simulink model "AxialPump_23a"  (R2023a)
settings: Solver=FixedStepAuto  StartTime=0.0  StopTime=t_cycle  FixedStep=1e-8  RelTol=1e-3  EnableMultiTasking=on
InitFcn:
  | %% Outlet
  | % Parameters
  | d_cyl = 8e-3;                                   % Diameter of each piston
  | r_p = 20e-3;                                    % Piston pitch radius
  | A_cyl = 0.25 * pi * d_cyl^2;                    % Area of each piston
  | omega_rpm = 3600;                               % Rotational speed of pump
  | omega = (2*pi/60) * omega_rpm;                  % Angular speed of pump
  | beta = 1.6e9;                                   % Bulk Modulus
  | P1 = 21e6;                                      % Outlet pressure
  | S = 15e-3;                                      % Stroke length
  | Cd = 0.6;                                       % Coefficient of discharge
  | rho = 870;                                      % Density
  | P_T = 101325;                                   % Tank pressure
  | P_P = 21e6;                                     % System pressure
  | c = 80e-6;                                      % Piston-barrel clearance
  | meu = 0.1;                                      % Steel-steel (lubricated) coefficient of friction
  | r2_r1 = 1.6;                                    % Slipper radii ratio
  | r1 = d_cyl/2;
  | do = 0.1e-3;                                    % Slipper orifice opening
  | 
  | % Time parameters
  | theta_cycle = 2 * pi;
  | t_cycle = theta_cycle / omega;
  | theta_t = 2 * asin(d_cyl/(4*r_p));
  | t_t = theta_t/omega;
  | theta_d = theta_cycle/2 - 2 * theta_t;
  | t_d = theta_d/omega;
  | 
  | t_A_p = [0, 0.5*t_t, t_t, t_t+t_d, 1.5*t_t+t_d, t_cycle];
  | A_p = [0, 0, A_cyl, A_cyl, 0, 0];
  | 
  | t_A_t = [0, 2.5*t_t+t_d, 3*t_t+t_d, 3*t_t+2*t_d, 3.5*t_t+2*t_d, t_cycle];
  | A_t = [0, 0, A_cyl, A_cyl, 0, 0];
  | 
  | % Calculated parameters
  | Vdisp = 0.25 * pi * d_cyl^2 * S;
  | Vo = Vdisp;
libraries: SignalEditorBlockLib x18
(part 1 of 2)
settings Model: Creator=user  LastModifiedBy=ibrah408
settings SolverCC: AutoInsertRateTranBlk=on
settings DataIOCC: SaveOutput=off  SaveTime=off
settings OptimizationCC: DefaultParameterBehavior=Inlined  InlineInvariantSignals=on  EnhancedBackFolding=on  PassReuseOutputArgsAs=Individual arguments  StateBitsets=on  DataBitsets=on  ZeroExternalMemoryAtStartup=off  ZeroInternalMemoryAtStartup=off  NoFixptDivByZeroProtection=on  LifeSpan=1  OptimizeBlockOrder=speed  DifferentSizesBufferReuse=on  EfficientTunableParamExpr=on
settings DebuggingCC: ParameterTunabilityLossMsg=error
settings HardwareCC: ProdBitPerPointer=32  ProdBitPerSizeT=32  ProdBitPerPtrDiffT=32  ProdLargestAtomicFloat=None  ProdIntDivRoundTo=Floor  ProdWordSize=32  ProdHWDeviceType=Generic->Custom
settings SFSimCC: MATLABDynamicMemAlloc=off
settings RTWCC: Description=Embedded Coder  SystemTargetFile=ert.tlc  TLCOptions=-p0  GenCodeOnly=on  TemplateMakefile=ert_default_tmf  GenerateReport=on  RTWVerbose=off  IncludeHyperlinkInReport=on  LaunchReport=on
settings CodeAppCC: ForceParamTrailComments=on  IgnoreCustomStorageClasses=off  OperatorAnnotations=on  SimulinkDataObjDesc=on  SFDataObjDesc=on  CustomSymbolStrGlobalVar=rt$N$M  CustomSymbolStrType=$N$M  CustomSymbolStrFcn=$N$M$F  CustomSymbolStrMacro=$N$M  InsertBlockDesc=on
settings ERTTargetCC: TargetLangStandard=C99 (ISO)  CodeReplacementLibrary=ISO_C  GenerateSampleERTMain=on  IncludeMdlTerminateFcn=off  SuppressErrorStatus=on  SupportAbsoluteTime=off  PurelyIntegerCode=on  SupportNonFinite=off  SupportComplex=off  InlinedParameterPlacement=NonHierarchical  RootIOFormat=Structure reference  ERTCustomFileTemplate=example_file_process.tlc

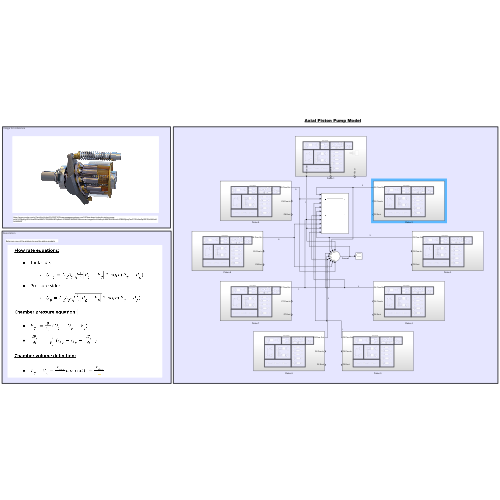
[thumbnail: Simulink's stored preview of the top-level diagram]
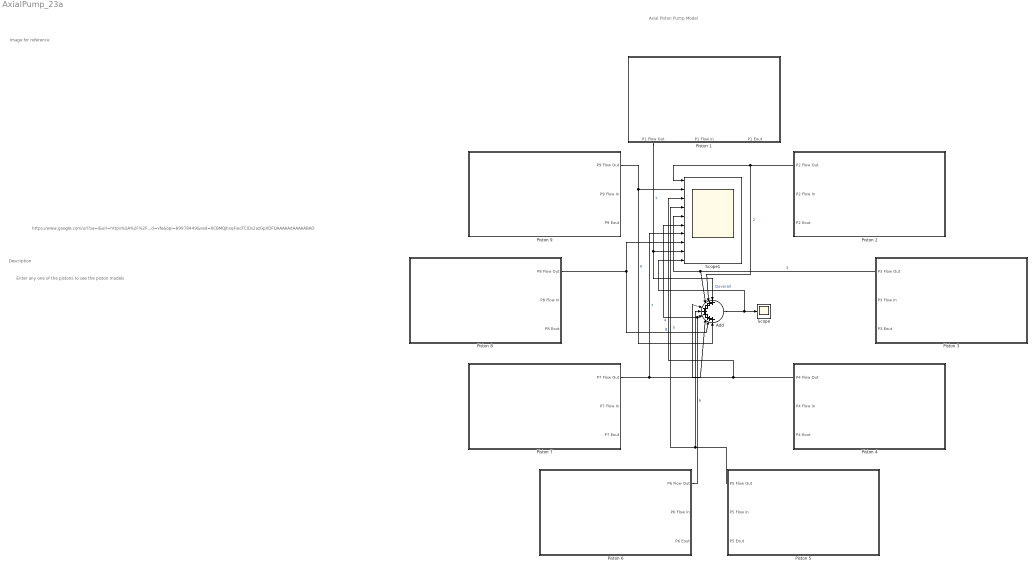
== system AxialPump_23a ==
  note: https://www.google.com/url?sa=i&url=https%3A%2F%2Fwww.panagonsystems.com%2Fhow-does-hydraulic-piston-pump-work%2F&psig=AOvVaw3SHzdt8MCUTcQAiBkLNfYq&ust=1698988184504000&source=images&cd=vfe&opi=89978449&ved=0CBMQjhxqFwoTCIDs2azGpIIDFQAAAAAdAAAAABAD
  note: Enter any one of the pistons to see the piston models
  note: Description
  note: Image for reference
  note: Axial Piston Pump Model
  Add : Sum  Inputs=+++++++++
  Piston 1 : Subsystem
      settings: PortSchema="{\"entries\":[{\"content\":{\"sides\":[{\"content\":{},\"type\":\"ConnectorPlacement.EquallySpacedRectSide\",\"uuid\":\"63442bf7-0830-4237-9a0b-f9adcef68f77\"},{\"content\":{\"side\":\"RIGHT\"},\"type\":\"ConnectorPlacement.EquallySpacedRectSide\",\"uuid\":\"c78b6823-6588-400d-8e0d-405a7015a902\"},{\"content\":{\"side\":\"TOP\"},\"type\":\"ConnectorPlacement.EquallySpacedRectSide\",\"uuid\":\"cf447a47-df1d-44f3-9a90-4edf3edff747\"},{\"content\":{\"connectorIds\":[\"Out1\",\"Out2\",\"Out3\"],\"side\":\"BOTTOM\"},\"type\":\"ConnectorPlacement.EquallySpacedRectSide\",\"uuid\":\"be505e56-dc88-4cf5-89cd-0d030a778f3c\"}]},\"type\":\"ConnectorPlacement.EquallySpacedConnector\",\"uuid\":\"51a26e02-629a-4264-944b-dee0710ca6c7\"}],\"packageUris\":[\"http://schema.mathworks.com/mf0/Connector/R2020b\"],\"version\":\"1.0\"}"
  Piston 2 : Subsystem
  Piston 3 : Subsystem
  Piston 4 : Subsystem
  Piston 5 : Subsystem
  Piston 6 : Subsystem
  Piston 7 : Subsystem
  Piston 8 : Subsystem
  Piston 9 : Subsystem
  Scope : Scope
  Scope1 : Scope  NumInputPorts=10
  wires:
  Add/1 -> Scope1/10, Scope/1  "Qoverall"
  Piston 2/1(P2 Flow Out) -> Scope1/1, Add/2  "2"
  Piston 3/1(P3 Flow Out) -> Scope1/5, Add/3  "3"
  Piston 4/1(P4 Flow Out) -> Scope1/3, Add/4  "4"
  Piston 5/1(P5 Flow Out) -> Add/5, Scope1/4  "5"
  Piston 6/1(P6 Flow Out) -> Scope1/6, Add/6  "6"
  Piston 7/1(P7 Flow Out) -> Scope1/7, Add/7  "7"
  Piston 8/1(P8 Flow Out) -> Add/8, Scope1/8  "8"
  Piston 9/1(P9 Flow Out) -> Add/9, Scope1/2  "9"
  Piston 1/1(P1 Flow Out) -> Add/1, Scope1/9  "1"

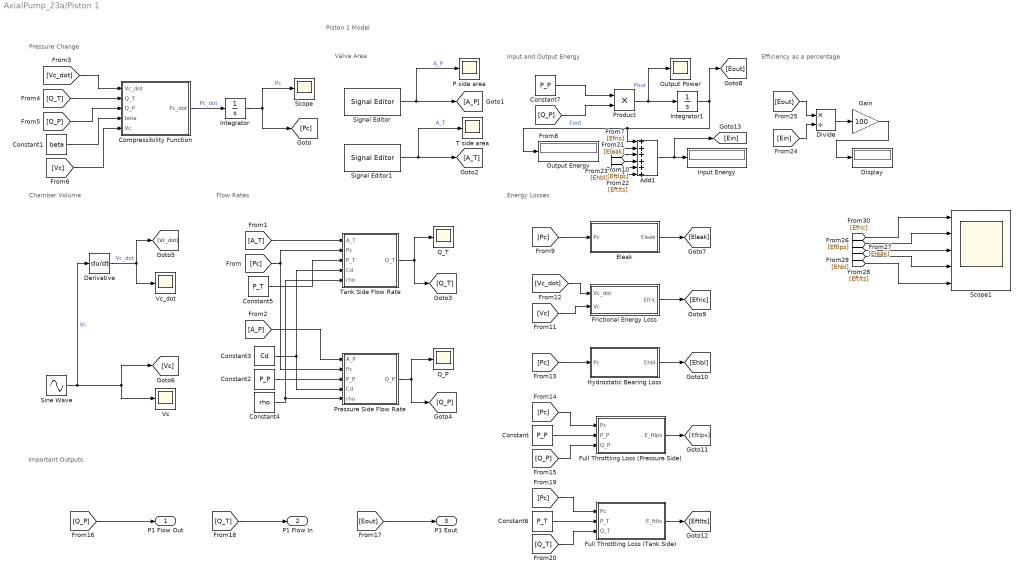
== system AxialPump_23a/Piston 1 ==
  note: Efficiency as a percentage
  note: Important Outputs
  note: Energy Losses
  note: Input and Output Energy
  note: Pressure Change
  note: Chamber Volume
  note: Valve Area
  note: Flow Rates
  note: Piston 1 Model
      | ​
  Add1 : Sum  Inputs=++++++
  Compressibility Function : MATLAB Function  TreatAsAtomicUnit=on
  Constant : Constant  Value=P_P
  Constant1 : Constant  Value=beta
  Constant2 : Constant  Value=P_P
  Constant3 : Constant  Value=Cd
  Constant4 : Constant  Value=rho
  Constant5 : Constant  Value=P_T
  Constant6 : Constant  Value=P_T
  Constant7 : Constant  Value=P_P
  Derivative : Derivative
  Display : Display
  Divide : Product  Inputs=*/
  Eleak : Subsystem
  Frictional Energy Loss : Subsystem
  Full Throttling Loss (Pressure Side) : Subsystem
  Full Throttling Loss (Tank Side) : Subsystem
  Gain : Gain  Gain=100
  Hydrostatic Bearing Loss : Subsystem
  Input Energy : Display
  Integrator : Integrator  InitialCondition=-2.0291e6  LowerSaturationLimit=0
  Integrator1 : Integrator
  Output Energy : Display
  Output Power : Scope
  P side area : Scope
  Pressure Side Flow Rate : MATLAB Function  TreatAsAtomicUnit=on
  Product : Product
  Q_P : Scope
  Q_T : Scope
  Scope : Scope
  Scope1 : Scope  NumInputPorts=5
  Signal Editor : SignalEditorBlockLib/Signal Editor  FileName=A_P.mat  ActiveScenario=Scenario  ActiveSignal=A_P  IsBus=off  OutputBusObjectStr=Bus: BusObject  SampleTime=0  ZeroCross=off  OutputAfterFinalValue=Setting to zero  Unit=inherit  PreserveSignalName=on  ApplySigPropsToAllScenarios=on
  Signal Editor1 : SignalEditorBlockLib/Signal Editor  FileName=A_T.mat  ActiveScenario=Scenario  ActiveSignal=A_T  IsBus=off  OutputBusObjectStr=Bus: BusObject  SampleTime=0  ZeroCross=off  OutputAfterFinalValue=Setting to zero  Unit=inherit  PreserveSignalName=on  ApplySigPropsToAllScenarios=on
  Sine Wave : Sin  Amplitude=Vdisp/2  Bias=Vo + (Vdisp/2)  Frequency=omega  Phase=pi/2  SampleTime=0
  T side area : Scope
  Tank Side Flow Rate : MATLAB Function  TreatAsAtomicUnit=on
  Vc : Scope
  Vc_dot : Scope
  P1 Flow Out : Outport
  P1 Flow In : Outport  Port=2
  P1 Eout : Outport  Port=3
  wires:
  Signal Editor/1 -> P side area/1, [A_P]  "A_P"
  [Pc] -> Hydrostatic Bearing Loss/1(Pc)
  [A_P] -> Pressure Side Flow Rate/1(A_P)
  [Pc] -> Full Throttling Loss (Pressure Side)/1(Pc)
  [Q_P] -> Full Throttling Loss (Pressure Side)/3(Q_P)
  Constant/1 -> Full Throttling Loss (Pressure Side)/2(P_P)
  Pressure Side Flow Rate/1(Q_P) -> Q_P/1, [Q_P]
  Tank Side Flow Rate/1(Q_T) -> Q_T/1, [Q_T]
  Constant4/1 -> Tank Side Flow Rate/5(rho), Pressure Side Flow Rate/5(rho)
  Constant2/1 -> Pressure Side Flow Rate/3(P_P)
  [Q_P] -> Compressibility Function/3(Q_P)
  Signal Editor1/1 -> [A_T], T side area/1  "A_T"
  [A_T] -> Tank Side Flow Rate/1(A_T)
  Constant1/1 -> Compressibility Function/4(beta)
  [Pc] -> Pressure Side Flow Rate/2(Pc), Tank Side Flow Rate/2(Pc)
  [Vc_dot] -> Compressibility Function/1(Vc_dot)
  [Q_T] -> Compressibility Function/2(Q_T)
  Compressibility Function/1(Pc_dot) -> Integrator/1  "Pc_dot"
  [Vc] -> Compressibility Function/5(Vc)
  Sine Wave/1 -> [Vc], Vc/1, Derivative/1  "Vc"
  Integrator/1 -> [Pc], Scope/1  "Pc"
  Constant3/1 -> Tank Side Flow Rate/4(Cd), Pressure Side Flow Rate/4(Cd)
  Derivative/1 -> Vc_dot/1, [Vc_dot]  "Vc_dot"
  Constant5/1 -> Tank Side Flow Rate/3(P_T)
  [Vc_dot] -> Frictional Energy Loss/1(Vc_dot)
  [Vc] -> Frictional Energy Loss/2(Vc)
  [Q_P] -> P1 Flow Out/1
  [Eout] -> P1 Eout/1
  [Q_T] -> P1 Flow In/1
  [Pc] -> Full Throttling Loss (Tank Side)/1(Pc)
  Constant6/1 -> Full Throttling Loss (Tank Side)/2(P_T)
  [Q_T] -> Full Throttling Loss (Tank Side)/3(Q_T)
  Constant7/1 -> Product/1
  Product/1 -> Integrator1/1, Output Power/1  "Pout"
  Add1/1 -> [Ein], Input Energy/1
  Integrator1/1 -> Output Energy/1, Add1/1, [Eout]  "Eout"
  [Q_P] -> Product/2
  [Pc] -> Eleak/1(Pc)
  Eleak/1(Eleak) -> [Eleak]
  Frictional Energy Loss/1(Efric) -> [Efric]
  Hydrostatic Bearing Loss/1(Ehbl) -> [Ehbl]
  Full Throttling Loss (Tank Side)/1(" E_ftlts") -> [Eftlts]
  Full Throttling Loss (Pressure Side)/1(" E_ftlps") -> [Eftlps]
  [Efric] -> Add1/2
  [Eftlps] -> Add1/3
  [Eleak] -> Add1/4
  [Eftlts] -> Add1/5
  [Ehbl] -> Add1/6
  [Ein] -> Divide/2
  [Eout] -> Divide/1
  Divide/1 -> Gain/1
  Gain/1 -> Display/1
  [Efric] -> Scope1/1
  [Eftlps] -> Scope1/2
  [Eleak] -> Scope1/3
  [Eftlts] -> Scope1/4
  [Ehbl] -> Scope1/5

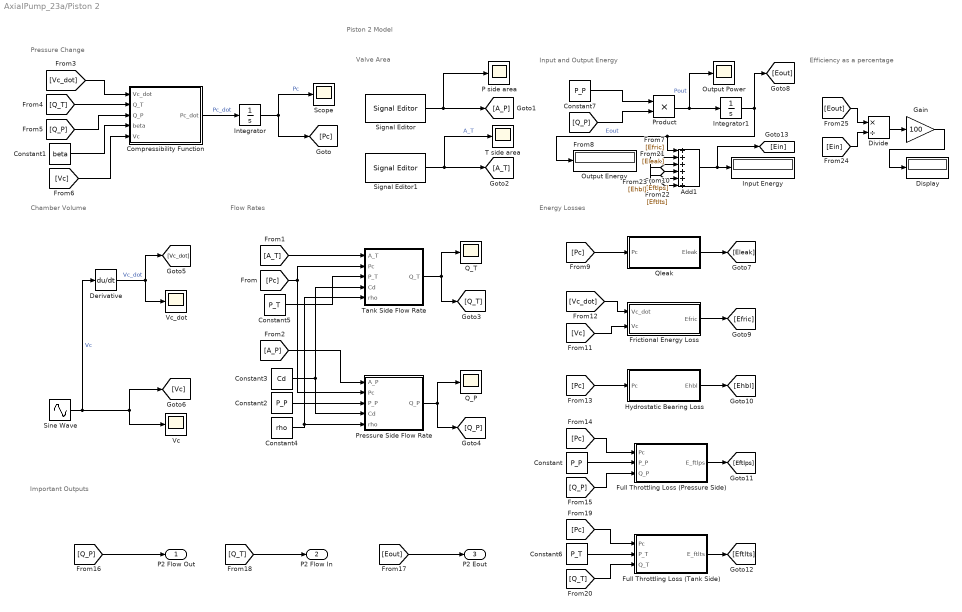
== system AxialPump_23a/Piston 2 ==
  note: Important Outputs
  note: Pressure Change
  note: Chamber Volume
  note: Valve Area
  note: Flow Rates
  note: Piston 2 Model
      | ​
  note: Energy Losses
  note: Efficiency as a percentage
  note: Input and Output Energy
  Add1 : Sum  Inputs=++++++
  Compressibility Function : MATLAB Function  TreatAsAtomicUnit=on
  Constant : Constant  Value=P_P
  Constant1 : Constant  Value=beta
  Constant2 : Constant  Value=P_P
  Constant3 : Constant  Value=Cd
  Constant4 : Constant  Value=rho
  Constant5 : Constant  Value=P_T
  Constant6 : Constant  Value=P_T
  Constant7 : Constant  Value=P_P
  Derivative : Derivative
  Display : Display
  Divide : Product  Inputs=*/
  Frictional Energy Loss : Subsystem
  Full Throttling Loss (Pressure Side) : Subsystem
  Full Throttling Loss (Tank Side) : Subsystem
  Gain : Gain  Gain=100
  Hydrostatic Bearing Loss : Subsystem
  Input Energy : Display
  Integrator : Integrator  InitialCondition=P_T
  Integrator1 : Integrator
  Output Energy : Display
  Output Power : Scope
  P side area : Scope
  Pressure Side Flow Rate : MATLAB Function  TreatAsAtomicUnit=on
  Product : Product
  Q_P : Scope
  Q_T : Scope
  Qleak : Subsystem
  Scope : Scope
  Signal Editor : SignalEditorBlockLib/Signal Editor  FileName=A_P_2.mat  ActiveScenario=Scenario  ActiveSignal=A_P_2  IsBus=off  OutputBusObjectStr=Bus: BusObject  SampleTime=0  ZeroCross=off  OutputAfterFinalValue=Setting to zero  Unit=inherit  PreserveSignalName=on  ApplySigPropsToAllScenarios=on
  Signal Editor1 : SignalEditorBlockLib/Signal Editor  FileName=A_T_2.mat  ActiveScenario=Scenario  ActiveSignal=A_T_2  IsBus=off  OutputBusObjectStr=Bus: BusObject  SampleTime=0  ZeroCross=off  OutputAfterFinalValue=Setting to zero  Unit=inherit  PreserveSignalName=on  ApplySigPropsToAllScenarios=on
  Sine Wave : Sin  Amplitude=Vdisp/2  Bias=Vo + (Vdisp/2)  Frequency=omega  Phase=pi/2-(2*pi/9)  SampleTime=0
  T side area : Scope
  Tank Side Flow Rate : MATLAB Function  TreatAsAtomicUnit=on
  Vc : Scope
  Vc_dot : Scope
  P2 Flow Out : Outport
  P2 Flow In : Outport  Port=2
  P2 Eout : Outport  Port=3
  wires:
  Signal Editor/1 -> P side area/1, [A_P]
  [A_P] -> Pressure Side Flow Rate/1(A_P)
  Pressure Side Flow Rate/1(Q_P) -> Q_P/1, [Q_P]
  Tank Side Flow Rate/1(Q_T) -> Q_T/1, [Q_T]
  Constant4/1 -> Tank Side Flow Rate/5(rho), Pressure Side Flow Rate/5(rho)
  Constant2/1 -> Pressure Side Flow Rate/3(P_P)
  [Q_P] -> Compressibility Function/3(Q_P)
  Signal Editor1/1 -> [A_T], T side area/1  "A_T"
  [A_T] -> Tank Side Flow Rate/1(A_T)
  Constant1/1 -> Compressibility Function/4(beta)
  [Pc] -> Pressure Side Flow Rate/2(Pc), Tank Side Flow Rate/2(Pc)
  [Vc_dot] -> Compressibility Function/1(Vc_dot)
  [Q_T] -> Compressibility Function/2(Q_T)
  Compressibility Function/1(Pc_dot) -> Integrator/1  "Pc_dot"
  [Vc] -> Compressibility Function/5(Vc)
  Sine Wave/1 -> [Vc], Vc/1, Derivative/1  "Vc"
  Integrator/1 -> [Pc], Scope/1  "Pc"
  Constant3/1 -> Tank Side Flow Rate/4(Cd), Pressure Side Flow Rate/4(Cd)
  Derivative/1 -> Vc_dot/1, [Vc_dot]  "Vc_dot"
  Constant5/1 -> Tank Side Flow Rate/3(P_T)
  [Q_P] -> P2 Flow Out/1
  [Eout] -> P2 Eout/1
  [Q_T] -> P2 Flow In/1
  [Pc] -> Qleak/1(Pc)
  [Eout] -> Divide/1
  Full Throttling Loss (Pressure Side)/1(" E_ftlps") -> [Eftlps]
  Full Throttling Loss (Tank Side)/1(" E_ftlts") -> [Eftlts]
  [Eftlts] -> Add1/5
  [Ehbl] -> Add1/6
  [Q_T] -> Full Throttling Loss (Tank Side)/3(Q_T)
  [Pc] -> Full Throttling Loss (Pressure Side)/1(Pc)
  [Pc] -> Full Throttling Loss (Tank Side)/1(Pc)
  [Vc] -> Frictional Energy Loss/2(Vc)
  [Vc_dot] -> Frictional Energy Loss/1(Vc_dot)
  [Pc] -> Hydrostatic Bearing Loss/1(Pc)
  Constant/1 -> Full Throttling Loss (Pressure Side)/2(P_P)
  [Q_P] -> Full Throttling Loss (Pressure Side)/3(Q_P)
  [Q_P] -> Product/2
  [Efric] -> Add1/2
  Constant6/1 -> Full Throttling Loss (Tank Side)/2(P_T)
  [Ein] -> Divide/2
  Divide/1 -> Gain/1
  Frictional Energy Loss/1(Efric) -> [Efric]
  Product/1 -> Integrator1/1, Output Power/1  "Pout"
  Constant7/1 -> Product/1
  Hydrostatic Bearing Loss/1(Ehbl) -> [Ehbl]
  Gain/1 -> Display/1
  Qleak/1(Eleak) -> [Eleak]
  Integrator1/1 -> Output Energy/1, Add1/1, [Eout]  "Eout"
  [Eftlps] -> Add1/3
  [Eleak] -> Add1/4
  Add1/1 -> [Ein], Input Energy/1

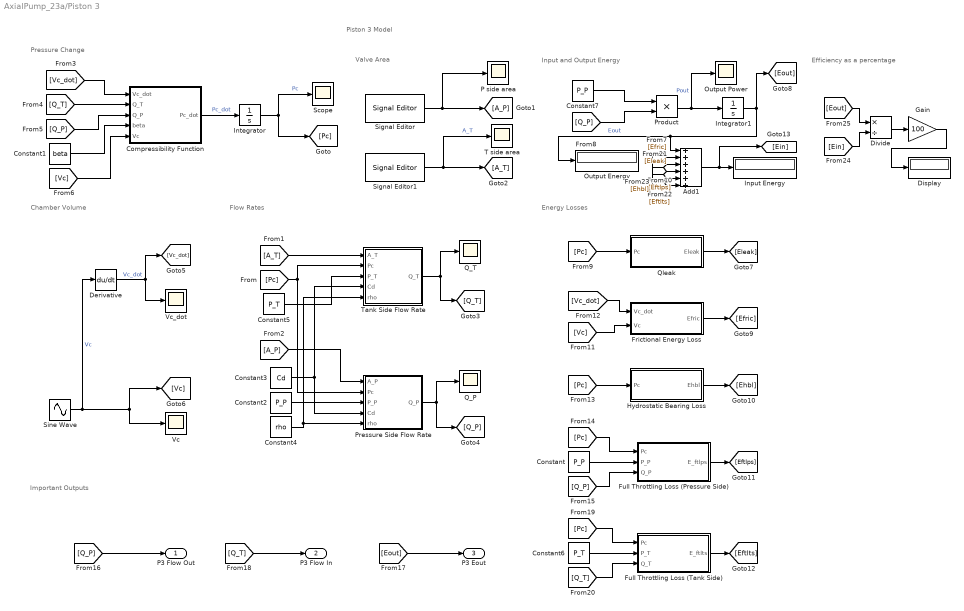
== system AxialPump_23a/Piston 3 ==
  note: Important Outputs
  note: Pressure Change
  note: Chamber Volume
  note: Valve Area
  note: Flow Rates
  note: Piston 3 Model
      | ​
  note: Energy Losses
  note: Efficiency as a percentage
  note: Input and Output Energy
  Add1 : Sum  Inputs=++++++
  Compressibility Function : MATLAB Function  TreatAsAtomicUnit=on
  Constant : Constant  Value=P_P
  Constant1 : Constant  Value=beta
  Constant2 : Constant  Value=P_P
  Constant3 : Constant  Value=Cd
  Constant4 : Constant  Value=rho
  Constant5 : Constant  Value=P_T
  Constant6 : Constant  Value=P_T
  Constant7 : Constant  Value=P_P
  Derivative : Derivative
  Display : Display
  Divide : Product  Inputs=*/
  Frictional Energy Loss : Subsystem
  Full Throttling Loss (Pressure Side) : Subsystem
  Full Throttling Loss (Tank Side) : Subsystem
  Gain : Gain  Gain=100
  Hydrostatic Bearing Loss : Subsystem
  Input Energy : Display
  Integrator : Integrator  InitialCondition=P_T
  Integrator1 : Integrator
  Output Energy : Display
  Output Power : Scope
  P side area : Scope
  Pressure Side Flow Rate : MATLAB Function  TreatAsAtomicUnit=on
  Product : Product
  Q_P : Scope
  Q_T : Scope
  Qleak : Subsystem
  Scope : Scope
  Signal Editor : SignalEditorBlockLib/Signal Editor  FileName=A_P_3.mat  ActiveScenario=Scenario  ActiveSignal=A_P_3  IsBus=off  OutputBusObjectStr=Bus: BusObject  SampleTime=0  ZeroCross=off  OutputAfterFinalValue=Setting to zero  Unit=inherit  PreserveSignalName=on  ApplySigPropsToAllScenarios=on
  Signal Editor1 : SignalEditorBlockLib/Signal Editor  FileName=A_T_3.mat  ActiveScenario=Scenario  ActiveSignal=A_T_3  IsBus=off  OutputBusObjectStr=Bus: BusObject  SampleTime=0  ZeroCross=off  OutputAfterFinalValue=Setting to zero  Unit=inherit  PreserveSignalName=on  ApplySigPropsToAllScenarios=on
  Sine Wave : Sin  Amplitude=Vdisp/2  Bias=Vo + (Vdisp/2)  Frequency=omega  Phase=pi/2-(4*pi/9)  SampleTime=0
  T side area : Scope
  Tank Side Flow Rate : MATLAB Function  TreatAsAtomicUnit=on
  Vc : Scope
  Vc_dot : Scope
  P3 Flow Out : Outport
  P3 Flow In : Outport  Port=2
  P3 Eout : Outport  Port=3
  wires:
  Signal Editor/1 -> P side area/1, [A_P]
  [A_P] -> Pressure Side Flow Rate/1(A_P)
  Pressure Side Flow Rate/1(Q_P) -> Q_P/1, [Q_P]
  Tank Side Flow Rate/1(Q_T) -> Q_T/1, [Q_T]
  Constant4/1 -> Tank Side Flow Rate/5(rho), Pressure Side Flow Rate/5(rho)
  Constant2/1 -> Pressure Side Flow Rate/3(P_P)
  [Q_P] -> Compressibility Function/3(Q_P)
  Signal Editor1/1 -> [A_T], T side area/1  "A_T"
  [A_T] -> Tank Side Flow Rate/1(A_T)
  Constant1/1 -> Compressibility Function/4(beta)
  [Pc] -> Pressure Side Flow Rate/2(Pc), Tank Side Flow Rate/2(Pc)
  [Vc_dot] -> Compressibility Function/1(Vc_dot)
  [Q_T] -> Compressibility Function/2(Q_T)
  Compressibility Function/1(Pc_dot) -> Integrator/1  "Pc_dot"
  [Vc] -> Compressibility Function/5(Vc)
  Sine Wave/1 -> [Vc], Vc/1, Derivative/1  "Vc"
  Integrator/1 -> [Pc], Scope/1  "Pc"
  Constant3/1 -> Tank Side Flow Rate/4(Cd), Pressure Side Flow Rate/4(Cd)
  Derivative/1 -> Vc_dot/1, [Vc_dot]  "Vc_dot"
  Constant5/1 -> Tank Side Flow Rate/3(P_T)
  [Q_P] -> P3 Flow Out/1
  [Eout] -> P3 Eout/1
  [Q_T] -> P3 Flow In/1
  [Pc] -> Qleak/1(Pc)
  [Eout] -> Divide/1
  Full Throttling Loss (Pressure Side)/1(" E_ftlps") -> [Eftlps]
  Full Throttling Loss (Tank Side)/1(" E_ftlts") -> [Eftlts]
  [Eftlts] -> Add1/5
  [Ehbl] -> Add1/6
  [Q_T] -> Full Throttling Loss (Tank Side)/3(Q_T)
  [Pc] -> Full Throttling Loss (Pressure Side)/1(Pc)
  [Pc] -> Full Throttling Loss (Tank Side)/1(Pc)
  [Vc] -> Frictional Energy Loss/2(Vc)
  [Vc_dot] -> Frictional Energy Loss/1(Vc_dot)
  [Pc] -> Hydrostatic Bearing Loss/1(Pc)
  Constant/1 -> Full Throttling Loss (Pressure Side)/2(P_P)
  [Q_P] -> Full Throttling Loss (Pressure Side)/3(Q_P)
  [Q_P] -> Product/2
  [Efric] -> Add1/2
  Constant6/1 -> Full Throttling Loss (Tank Side)/2(P_T)
  [Ein] -> Divide/2
  Divide/1 -> Gain/1
  Frictional Energy Loss/1(Efric) -> [Efric]
  Product/1 -> Integrator1/1, Output Power/1  "Pout"
  Constant7/1 -> Product/1
  Hydrostatic Bearing Loss/1(Ehbl) -> [Ehbl]
  Gain/1 -> Display/1
  Qleak/1(Eleak) -> [Eleak]
  Integrator1/1 -> Output Energy/1, Add1/1, [Eout]  "Eout"
  [Eftlps] -> Add1/3
  [Eleak] -> Add1/4
  Add1/1 -> [Ein], Input Energy/1

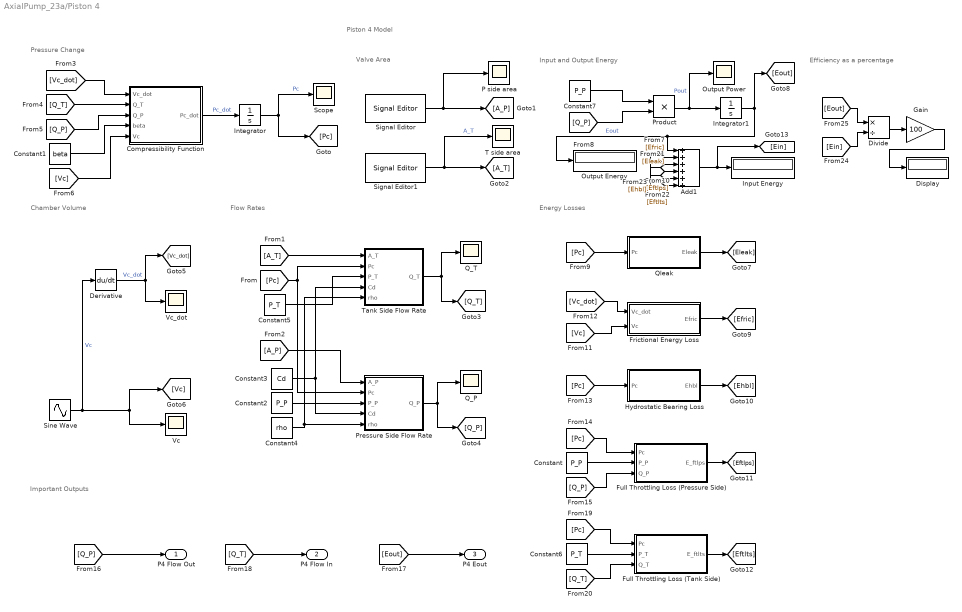
== system AxialPump_23a/Piston 4 ==
  note: Important Outputs
  note: Pressure Change
  note: Chamber Volume
  note: Valve Area
  note: Flow Rates
  note: Piston 4 Model
      | ​
  note: Energy Losses
  note: Efficiency as a percentage
  note: Input and Output Energy
  Add1 : Sum  Inputs=++++++
  Compressibility Function : MATLAB Function  TreatAsAtomicUnit=on
  Constant : Constant  Value=P_P
  Constant1 : Constant  Value=beta
  Constant2 : Constant  Value=P_P
  Constant3 : Constant  Value=Cd
  Constant4 : Constant  Value=rho
  Constant5 : Constant  Value=P_T
  Constant6 : Constant  Value=P_T
  Constant7 : Constant  Value=P_P
  Derivative : Derivative
  Display : Display
  Divide : Product  Inputs=*/
  Frictional Energy Loss : Subsystem
  Full Throttling Loss (Pressure Side) : Subsystem
  Full Throttling Loss (Tank Side) : Subsystem
  Gain : Gain  Gain=100
  Hydrostatic Bearing Loss : Subsystem
  Input Energy : Display
  Integrator : Integrator  InitialCondition=P_T
  Integrator1 : Integrator
  Output Energy : Display
  Output Power : Scope
  P side area : Scope
  Pressure Side Flow Rate : MATLAB Function  TreatAsAtomicUnit=on
  Product : Product
  Q_P : Scope
  Q_T : Scope
  Qleak : Subsystem
  Scope : Scope
  Signal Editor : SignalEditorBlockLib/Signal Editor  FileName=A_P_4.mat  ActiveScenario=Scenario  ActiveSignal=A_P_4  IsBus=off  OutputBusObjectStr=Bus: BusObject  SampleTime=0  ZeroCross=off  OutputAfterFinalValue=Setting to zero  Unit=inherit  PreserveSignalName=on  ApplySigPropsToAllScenarios=on
  Signal Editor1 : SignalEditorBlockLib/Signal Editor  FileName=A_T_4.mat  ActiveScenario=Scenario  ActiveSignal=A_T_4  IsBus=off  OutputBusObjectStr=Bus: BusObject  SampleTime=0  ZeroCross=off  OutputAfterFinalValue=Setting to zero  Unit=inherit  PreserveSignalName=on  ApplySigPropsToAllScenarios=on
  Sine Wave : Sin  Amplitude=Vdisp/2  Bias=Vo + (Vdisp/2)  Frequency=omega  Phase=pi/2-(6*pi/9)  SampleTime=0
  T side area : Scope
  Tank Side Flow Rate : MATLAB Function  TreatAsAtomicUnit=on
  Vc : Scope
  Vc_dot : Scope
  P4 Flow Out : Outport
  P4 Flow In : Outport  Port=2
  P4 Eout : Outport  Port=3
  wires:
  Signal Editor/1 -> P side area/1, [A_P]
  [A_P] -> Pressure Side Flow Rate/1(A_P)
  Pressure Side Flow Rate/1(Q_P) -> Q_P/1, [Q_P]
  Tank Side Flow Rate/1(Q_T) -> Q_T/1, [Q_T]
  Constant4/1 -> Tank Side Flow Rate/5(rho), Pressure Side Flow Rate/5(rho)
  Constant2/1 -> Pressure Side Flow Rate/3(P_P)
  [Q_P] -> Compressibility Function/3(Q_P)
  Signal Editor1/1 -> [A_T], T side area/1  "A_T"
  [A_T] -> Tank Side Flow Rate/1(A_T)
  Constant1/1 -> Compressibility Function/4(beta)
  [Pc] -> Pressure Side Flow Rate/2(Pc), Tank Side Flow Rate/2(Pc)
  [Vc_dot] -> Compressibility Function/1(Vc_dot)
  [Q_T] -> Compressibility Function/2(Q_T)
  Compressibility Function/1(Pc_dot) -> Integrator/1  "Pc_dot"
  [Vc] -> Compressibility Function/5(Vc)
  Sine Wave/1 -> [Vc], Vc/1, Derivative/1  "Vc"
  Integrator/1 -> [Pc], Scope/1  "Pc"
  Constant3/1 -> Tank Side Flow Rate/4(Cd), Pressure Side Flow Rate/4(Cd)
  Derivative/1 -> Vc_dot/1, [Vc_dot]  "Vc_dot"
  Constant5/1 -> Tank Side Flow Rate/3(P_T)
  [Q_P] -> P4 Flow Out/1
  [Eout] -> P4 Eout/1
  [Q_T] -> P4 Flow In/1
  [Pc] -> Qleak/1(Pc)
  [Eout] -> Divide/1
  Full Throttling Loss (Pressure Side)/1(" E_ftlps") -> [Eftlps]
  Full Throttling Loss (Tank Side)/1(" E_ftlts") -> [Eftlts]
  [Eftlts] -> Add1/5
  [Ehbl] -> Add1/6
  [Q_T] -> Full Throttling Loss (Tank Side)/3(Q_T)
  [Pc] -> Full Throttling Loss (Pressure Side)/1(Pc)
  [Pc] -> Full Throttling Loss (Tank Side)/1(Pc)
  [Vc] -> Frictional Energy Loss/2(Vc)
  [Vc_dot] -> Frictional Energy Loss/1(Vc_dot)
  [Pc] -> Hydrostatic Bearing Loss/1(Pc)
  Constant/1 -> Full Throttling Loss (Pressure Side)/2(P_P)
  [Q_P] -> Full Throttling Loss (Pressure Side)/3(Q_P)
  [Q_P] -> Product/2
  [Efric] -> Add1/2
  Constant6/1 -> Full Throttling Loss (Tank Side)/2(P_T)
  [Ein] -> Divide/2
  Divide/1 -> Gain/1
  Frictional Energy Loss/1(Efric) -> [Efric]
  Product/1 -> Integrator1/1, Output Power/1  "Pout"
  Constant7/1 -> Product/1
  Hydrostatic Bearing Loss/1(Ehbl) -> [Ehbl]
  Gain/1 -> Display/1
  Qleak/1(Eleak) -> [Eleak]
  Integrator1/1 -> Output Energy/1, Add1/1, [Eout]  "Eout"
  [Eftlps] -> Add1/3
  [Eleak] -> Add1/4
  Add1/1 -> [Ein], Input Energy/1

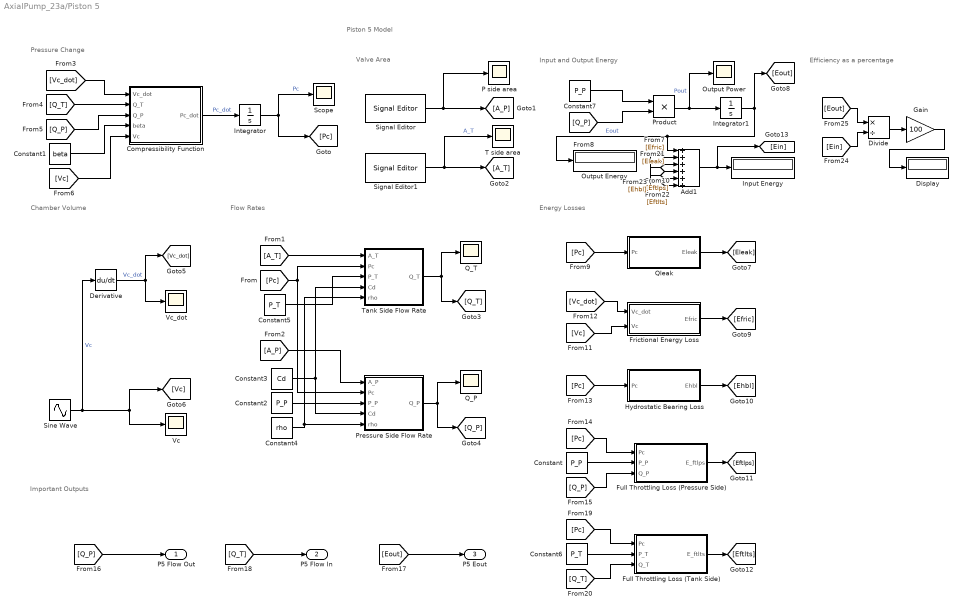
== system AxialPump_23a/Piston 5 ==
  note: Important Outputs
  note: Pressure Change
  note: Chamber Volume
  note: Valve Area
  note: Flow Rates
  note: Piston 5 Model
      | ​
  note: Energy Losses
  note: Efficiency as a percentage
  note: Input and Output Energy
  Add1 : Sum  Inputs=++++++
  Compressibility Function : MATLAB Function  TreatAsAtomicUnit=on
  Constant : Constant  Value=P_P
  Constant1 : Constant  Value=beta
  Constant2 : Constant  Value=P_P
  Constant3 : Constant  Value=Cd
  Constant4 : Constant  Value=rho
  Constant5 : Constant  Value=P_T
  Constant6 : Constant  Value=P_T
  Constant7 : Constant  Value=P_P
  Derivative : Derivative
  Display : Display
  Divide : Product  Inputs=*/
  Frictional Energy Loss : Subsystem
  Full Throttling Loss (Pressure Side) : Subsystem
  Full Throttling Loss (Tank Side) : Subsystem
  Gain : Gain  Gain=100
  Hydrostatic Bearing Loss : Subsystem
  Input Energy : Display
  Integrator : Integrator  InitialCondition=P_T
  Integrator1 : Integrator
  Output Energy : Display
  Output Power : Scope
  P side area : Scope
  Pressure Side Flow Rate : MATLAB Function  TreatAsAtomicUnit=on
  Product : Product
  Q_P : Scope
  Q_T : Scope
  Qleak : Subsystem
  Scope : Scope
  Signal Editor : SignalEditorBlockLib/Signal Editor  FileName=A_P_5.mat  ActiveScenario=Scenario  ActiveSignal=A_P_5  IsBus=off  OutputBusObjectStr=Bus: BusObject  SampleTime=0  ZeroCross=off  OutputAfterFinalValue=Setting to zero  Unit=inherit  PreserveSignalName=on  ApplySigPropsToAllScenarios=on
  Signal Editor1 : SignalEditorBlockLib/Signal Editor  FileName=A_T_5.mat  ActiveScenario=Scenario  ActiveSignal=A_T_5  IsBus=off  OutputBusObjectStr=Bus: BusObject  SampleTime=0  ZeroCross=off  OutputAfterFinalValue=Setting to zero  Unit=inherit  PreserveSignalName=on  ApplySigPropsToAllScenarios=on
  Sine Wave : Sin  Amplitude=Vdisp/2  Bias=Vo + (Vdisp/2)  Frequency=omega  Phase=pi/2-(8*pi/9)  SampleTime=0
  T side area : Scope
  Tank Side Flow Rate : MATLAB Function  TreatAsAtomicUnit=on
  Vc : Scope
  Vc_dot : Scope
  P5 Flow Out : Outport
  P5 Flow In : Outport  Port=2
  P5 Eout : Outport  Port=3
  wires:
  Signal Editor/1 -> P side area/1, [A_P]
  [A_P] -> Pressure Side Flow Rate/1(A_P)
  Pressure Side Flow Rate/1(Q_P) -> Q_P/1, [Q_P]
  Tank Side Flow Rate/1(Q_T) -> Q_T/1, [Q_T]
  Constant4/1 -> Tank Side Flow Rate/5(rho), Pressure Side Flow Rate/5(rho)
  Constant2/1 -> Pressure Side Flow Rate/3(P_P)
  [Q_P] -> Compressibility Function/3(Q_P)
  Signal Editor1/1 -> [A_T], T side area/1  "A_T"
  [A_T] -> Tank Side Flow Rate/1(A_T)
  Constant1/1 -> Compressibility Function/4(beta)
  [Pc] -> Pressure Side Flow Rate/2(Pc), Tank Side Flow Rate/2(Pc)
  [Vc_dot] -> Compressibility Function/1(Vc_dot)
  [Q_T] -> Compressibility Function/2(Q_T)
  Compressibility Function/1(Pc_dot) -> Integrator/1  "Pc_dot"
  [Vc] -> Compressibility Function/5(Vc)
  Sine Wave/1 -> [Vc], Vc/1, Derivative/1  "Vc"
  Integrator/1 -> [Pc], Scope/1  "Pc"
  Constant3/1 -> Tank Side Flow Rate/4(Cd), Pressure Side Flow Rate/4(Cd)
  Derivative/1 -> Vc_dot/1, [Vc_dot]  "Vc_dot"
  Constant5/1 -> Tank Side Flow Rate/3(P_T)
  [Q_P] -> P5 Flow Out/1
  [Eout] -> P5 Eout/1
  [Q_T] -> P5 Flow In/1
  [Pc] -> Qleak/1(Pc)
  [Eout] -> Divide/1
  Full Throttling Loss (Pressure Side)/1(" E_ftlps") -> [Eftlps]
  Full Throttling Loss (Tank Side)/1(" E_ftlts") -> [Eftlts]
  [Eftlts] -> Add1/5
  [Ehbl] -> Add1/6
  [Q_T] -> Full Throttling Loss (Tank Side)/3(Q_T)
  [Pc] -> Full Throttling Loss (Pressure Side)/1(Pc)
  [Pc] -> Full Throttling Loss (Tank Side)/1(Pc)
  [Vc] -> Frictional Energy Loss/2(Vc)
  [Vc_dot] -> Frictional Energy Loss/1(Vc_dot)
  [Pc] -> Hydrostatic Bearing Loss/1(Pc)
  Constant/1 -> Full Throttling Loss (Pressure Side)/2(P_P)
  [Q_P] -> Full Throttling Loss (Pressure Side)/3(Q_P)
  [Q_P] -> Product/2
  [Efric] -> Add1/2
  Constant6/1 -> Full Throttling Loss (Tank Side)/2(P_T)
  [Ein] -> Divide/2
  Divide/1 -> Gain/1
  Frictional Energy Loss/1(Efric) -> [Efric]
  Product/1 -> Integrator1/1, Output Power/1  "Pout"
  Constant7/1 -> Product/1
  Hydrostatic Bearing Loss/1(Ehbl) -> [Ehbl]
  Gain/1 -> Display/1
  Qleak/1(Eleak) -> [Eleak]
  Integrator1/1 -> Output Energy/1, Add1/1, [Eout]  "Eout"
  [Eftlps] -> Add1/3
  [Eleak] -> Add1/4
  Add1/1 -> [Ein], Input Energy/1

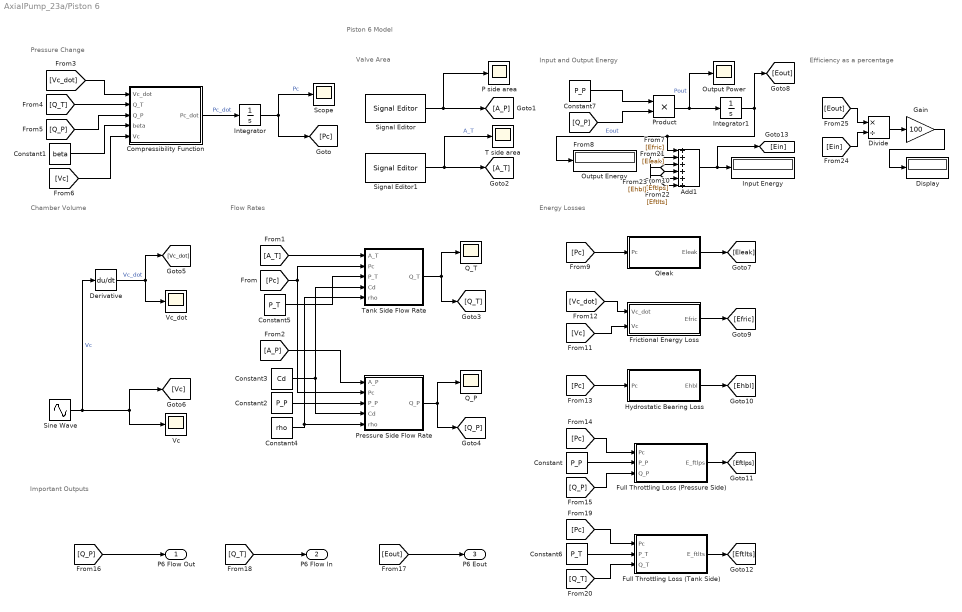
== system AxialPump_23a/Piston 6 ==
  note: Important Outputs
  note: Pressure Change
  note: Chamber Volume
  note: Valve Area
  note: Flow Rates
  note: Piston 6 Model
      | ​
  note: Energy Losses
  note: Efficiency as a percentage
  note: Input and Output Energy
  Add1 : Sum  Inputs=++++++
  Compressibility Function : MATLAB Function  TreatAsAtomicUnit=on
  Constant : Constant  Value=P_P
  Constant1 : Constant  Value=beta
  Constant2 : Constant  Value=P_P
  Constant3 : Constant  Value=Cd
  Constant4 : Constant  Value=rho
  Constant5 : Constant  Value=P_T
  Constant6 : Constant  Value=P_T
  Constant7 : Constant  Value=P_P
  Derivative : Derivative
  Display : Display
  Divide : Product  Inputs=*/
  Frictional Energy Loss : Subsystem
  Full Throttling Loss (Pressure Side) : Subsystem
  Full Throttling Loss (Tank Side) : Subsystem
  Gain : Gain  Gain=100
  Hydrostatic Bearing Loss : Subsystem
  Input Energy : Display
  Integrator : Integrator  InitialCondition=P_T
  Integrator1 : Integrator
  Output Energy : Display
  Output Power : Scope
  P side area : Scope
  Pressure Side Flow Rate : MATLAB Function  TreatAsAtomicUnit=on
  Product : Product
  Q_P : Scope
  Q_T : Scope
  Qleak : Subsystem
  Scope : Scope
  Signal Editor : SignalEditorBlockLib/Signal Editor  FileName=A_P_6.mat  ActiveScenario=Scenario  ActiveSignal=A_P_6  IsBus=off  OutputBusObjectStr=Bus: BusObject  SampleTime=0  ZeroCross=off  OutputAfterFinalValue=Setting to zero  Unit=inherit  PreserveSignalName=on  ApplySigPropsToAllScenarios=on
  Signal Editor1 : SignalEditorBlockLib/Signal Editor  FileName=A_T_6.mat  ActiveScenario=Scenario  ActiveSignal=A_T_6  IsBus=off  OutputBusObjectStr=Bus: BusObject  SampleTime=0  ZeroCross=off  OutputAfterFinalValue=Setting to zero  Unit=inherit  PreserveSignalName=on  ApplySigPropsToAllScenarios=on
  Sine Wave : Sin  Amplitude=Vdisp/2  Bias=Vo + (Vdisp/2)  Frequency=omega  Phase=pi/2-(10*pi/9)  SampleTime=0
  T side area : Scope
  Tank Side Flow Rate : MATLAB Function  TreatAsAtomicUnit=on
  Vc : Scope
  Vc_dot : Scope
  P6 Flow Out : Outport
  P6 Flow In : Outport  Port=2
  P6 Eout : Outport  Port=3
  wires:
  Signal Editor/1 -> P side area/1, [A_P]
  [A_P] -> Pressure Side Flow Rate/1(A_P)
  Pressure Side Flow Rate/1(Q_P) -> Q_P/1, [Q_P]
  Tank Side Flow Rate/1(Q_T) -> Q_T/1, [Q_T]
  Constant4/1 -> Tank Side Flow Rate/5(rho), Pressure Side Flow Rate/5(rho)
  Constant2/1 -> Pressure Side Flow Rate/3(P_P)
  [Q_P] -> Compressibility Function/3(Q_P)
  Signal Editor1/1 -> [A_T], T side area/1  "A_T"
  [A_T] -> Tank Side Flow Rate/1(A_T)
  Constant1/1 -> Compressibility Function/4(beta)
  [Pc] -> Pressure Side Flow Rate/2(Pc), Tank Side Flow Rate/2(Pc)
  [Vc_dot] -> Compressibility Function/1(Vc_dot)
  [Q_T] -> Compressibility Function/2(Q_T)
  Compressibility Function/1(Pc_dot) -> Integrator/1  "Pc_dot"
  [Vc] -> Compressibility Function/5(Vc)
  Sine Wave/1 -> [Vc], Vc/1, Derivative/1  "Vc"
  Integrator/1 -> [Pc], Scope/1  "Pc"
  Constant3/1 -> Tank Side Flow Rate/4(Cd), Pressure Side Flow Rate/4(Cd)
  Derivative/1 -> Vc_dot/1, [Vc_dot]  "Vc_dot"
  Constant5/1 -> Tank Side Flow Rate/3(P_T)
  [Q_P] -> P6 Flow Out/1
  [Eout] -> P6 Eout/1
  [Q_T] -> P6 Flow In/1
  [Pc] -> Qleak/1(Pc)
  [Eout] -> Divide/1
  Full Throttling Loss (Pressure Side)/1(" E_ftlps") -> [Eftlps]
  Full Throttling Loss (Tank Side)/1(" E_ftlts") -> [Eftlts]
  [Eftlts] -> Add1/5
  [Ehbl] -> Add1/6
  [Q_T] -> Full Throttling Loss (Tank Side)/3(Q_T)
  [Pc] -> Full Throttling Loss (Pressure Side)/1(Pc)
  [Pc] -> Full Throttling Loss (Tank Side)/1(Pc)
  [Vc] -> Frictional Energy Loss/2(Vc)
  [Vc_dot] -> Frictional Energy Loss/1(Vc_dot)
  [Pc] -> Hydrostatic Bearing Loss/1(Pc)
  Constant/1 -> Full Throttling Loss (Pressure Side)/2(P_P)
  [Q_P] -> Full Throttling Loss (Pressure Side)/3(Q_P)
  [Q_P] -> Product/2
  [Efric] -> Add1/2
  Constant6/1 -> Full Throttling Loss (Tank Side)/2(P_T)
  [Ein] -> Divide/2
  Divide/1 -> Gain/1
  Frictional Energy Loss/1(Efric) -> [Efric]
  Product/1 -> Integrator1/1, Output Power/1  "Pout"
  Constant7/1 -> Product/1
  Hydrostatic Bearing Loss/1(Ehbl) -> [Ehbl]
  Gain/1 -> Display/1
  Qleak/1(Eleak) -> [Eleak]
  Integrator1/1 -> Output Energy/1, Add1/1, [Eout]  "Eout"
  [Eftlps] -> Add1/3
  [Eleak] -> Add1/4
  Add1/1 -> [Ein], Input Energy/1

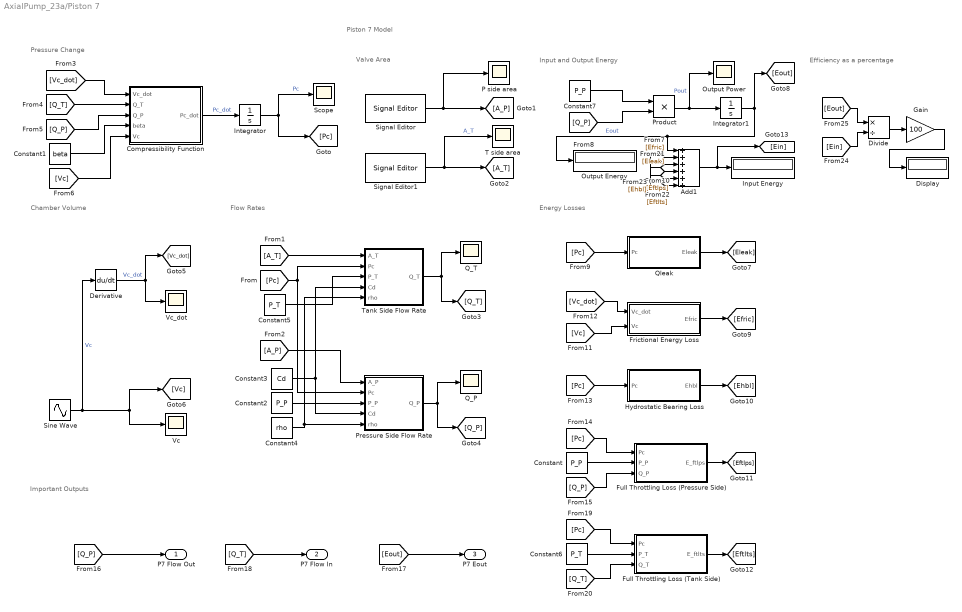
== system AxialPump_23a/Piston 7 ==
  note: Important Outputs
  note: Pressure Change
  note: Chamber Volume
  note: Valve Area
  note: Flow Rates
  note: Piston 7 Model
      | ​
  note: Energy Losses
  note: Efficiency as a percentage
  note: Input and Output Energy
  Add1 : Sum  Inputs=++++++
  Compressibility Function : MATLAB Function  TreatAsAtomicUnit=on
  Constant : Constant  Value=P_P
  Constant1 : Constant  Value=beta
  Constant2 : Constant  Value=P_P
  Constant3 : Constant  Value=Cd
  Constant4 : Constant  Value=rho
  Constant5 : Constant  Value=P_T
  Constant6 : Constant  Value=P_T
  Constant7 : Constant  Value=P_P
  Derivative : Derivative
  Display : Display
  Divide : Product  Inputs=*/
  Frictional Energy Loss : Subsystem
  Full Throttling Loss (Pressure Side) : Subsystem
  Full Throttling Loss (Tank Side) : Subsystem
  Gain : Gain  Gain=100
  Hydrostatic Bearing Loss : Subsystem
  Input Energy : Display
  Integrator : Integrator  InitialCondition=P_T
  Integrator1 : Integrator
  Output Energy : Display
  Output Power : Scope
  P side area : Scope
  Pressure Side Flow Rate : MATLAB Function  TreatAsAtomicUnit=on
  Product : Product
  Q_P : Scope
  Q_T : Scope
  Qleak : Subsystem
  Scope : Scope
  Signal Editor : SignalEditorBlockLib/Signal Editor  FileName=A_P_7.mat  ActiveScenario=Scenario  ActiveSignal=A_P_7  IsBus=off  OutputBusObjectStr=Bus: BusObject  SampleTime=0  ZeroCross=off  OutputAfterFinalValue=Setting to zero  Unit=inherit  PreserveSignalName=on  ApplySigPropsToAllScenarios=on
  Signal Editor1 : SignalEditorBlockLib/Signal Editor  FileName=A_T_7.mat  ActiveScenario=Scenario  ActiveSignal=A_T_7  IsBus=off  OutputBusObjectStr=Bus: BusObject  SampleTime=0  ZeroCross=off  OutputAfterFinalValue=Setting to zero  Unit=inherit  PreserveSignalName=on  ApplySigPropsToAllScenarios=on
  Sine Wave : Sin  Amplitude=Vdisp/2  Bias=Vo + (Vdisp/2)  Frequency=omega  Phase=pi/2-(12*pi/9)  SampleTime=0
  T side area : Scope
  Tank Side Flow Rate : MATLAB Function  TreatAsAtomicUnit=on
  Vc : Scope
  Vc_dot : Scope
  P7 Flow Out : Outport
  P7 Flow In : Outport  Port=2
  P7 Eout : Outport  Port=3
  wires:
  Signal Editor/1 -> P side area/1, [A_P]
  [A_P] -> Pressure Side Flow Rate/1(A_P)
  Pressure Side Flow Rate/1(Q_P) -> Q_P/1, [Q_P]
  Tank Side Flow Rate/1(Q_T) -> Q_T/1, [Q_T]
  Constant4/1 -> Tank Side Flow Rate/5(rho), Pressure Side Flow Rate/5(rho)
  Constant2/1 -> Pressure Side Flow Rate/3(P_P)
  [Q_P] -> Compressibility Function/3(Q_P)
  Signal Editor1/1 -> [A_T], T side area/1  "A_T"
  [A_T] -> Tank Side Flow Rate/1(A_T)
  Constant1/1 -> Compressibility Function/4(beta)
  [Pc] -> Pressure Side Flow Rate/2(Pc), Tank Side Flow Rate/2(Pc)
  [Vc_dot] -> Compressibility Function/1(Vc_dot)
  [Q_T] -> Compressibility Function/2(Q_T)
  Compressibility Function/1(Pc_dot) -> Integrator/1  "Pc_dot"
  [Vc] -> Compressibility Function/5(Vc)
  Sine Wave/1 -> [Vc], Vc/1, Derivative/1  "Vc"
  Integrator/1 -> [Pc], Scope/1  "Pc"
  Constant3/1 -> Tank Side Flow Rate/4(Cd), Pressure Side Flow Rate/4(Cd)
  Derivative/1 -> Vc_dot/1, [Vc_dot]  "Vc_dot"
  Constant5/1 -> Tank Side Flow Rate/3(P_T)
  [Q_P] -> P7 Flow Out/1
  [Eout] -> P7 Eout/1
  [Q_T] -> P7 Flow In/1
  [Pc] -> Qleak/1(Pc)
  [Eout] -> Divide/1
  Full Throttling Loss (Pressure Side)/1(" E_ftlps") -> [Eftlps]
  Full Throttling Loss (Tank Side)/1(" E_ftlts") -> [Eftlts]
  [Eftlts] -> Add1/5
  [Ehbl] -> Add1/6
  [Q_T] -> Full Throttling Loss (Tank Side)/3(Q_T)
  [Pc] -> Full Throttling Loss (Pressure Side)/1(Pc)
  [Pc] -> Full Throttling Loss (Tank Side)/1(Pc)
  [Vc] -> Frictional Energy Loss/2(Vc)
  [Vc_dot] -> Frictional Energy Loss/1(Vc_dot)
  [Pc] -> Hydrostatic Bearing Loss/1(Pc)
  Constant/1 -> Full Throttling Loss (Pressure Side)/2(P_P)
  [Q_P] -> Full Throttling Loss (Pressure Side)/3(Q_P)
  [Q_P] -> Product/2
  [Efric] -> Add1/2
  Constant6/1 -> Full Throttling Loss (Tank Side)/2(P_T)
  [Ein] -> Divide/2
  Divide/1 -> Gain/1
  Frictional Energy Loss/1(Efric) -> [Efric]
  Product/1 -> Integrator1/1, Output Power/1  "Pout"
  Constant7/1 -> Product/1
  Hydrostatic Bearing Loss/1(Ehbl) -> [Ehbl]
  Gain/1 -> Display/1
  Qleak/1(Eleak) -> [Eleak]
  Integrator1/1 -> Output Energy/1, Add1/1, [Eout]  "Eout"
  [Eftlps] -> Add1/3
  [Eleak] -> Add1/4
  Add1/1 -> [Ein], Input Energy/1

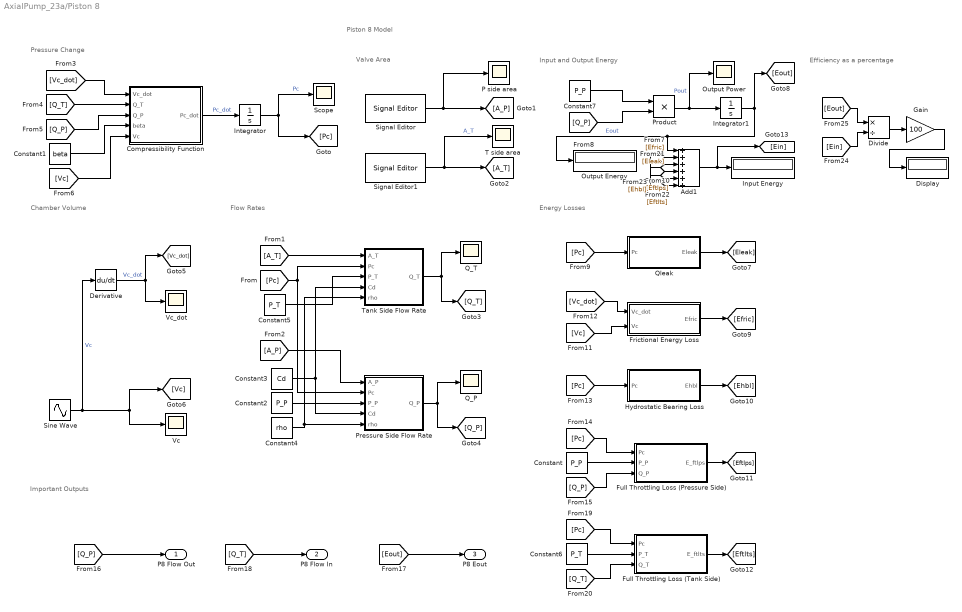
== system AxialPump_23a/Piston 8 ==
  note: Important Outputs
  note: Pressure Change
  note: Chamber Volume
  note: Valve Area
  note: Flow Rates
  note: Piston 8 Model
      | ​
  note: Energy Losses
  note: Efficiency as a percentage
  note: Input and Output Energy
  Add1 : Sum  Inputs=++++++
  Compressibility Function : MATLAB Function  TreatAsAtomicUnit=on
  Constant : Constant  Value=P_P
  Constant1 : Constant  Value=beta
  Constant2 : Constant  Value=P_P
  Constant3 : Constant  Value=Cd
  Constant4 : Constant  Value=rho
  Constant5 : Constant  Value=P_T
  Constant6 : Constant  Value=P_T
  Constant7 : Constant  Value=P_P
  Derivative : Derivative
  Display : Display
  Divide : Product  Inputs=*/
  Frictional Energy Loss : Subsystem
  Full Throttling Loss (Pressure Side) : Subsystem
  Full Throttling Loss (Tank Side) : Subsystem
  Gain : Gain  Gain=100
  Hydrostatic Bearing Loss : Subsystem
  Input Energy : Display
  Integrator : Integrator  InitialCondition=P_T
  Integrator1 : Integrator
  Output Energy : Display
  Output Power : Scope
  P side area : Scope
  Pressure Side Flow Rate : MATLAB Function  TreatAsAtomicUnit=on
  Product : Product
  Q_P : Scope
  Q_T : Scope
  Qleak : Subsystem
  Scope : Scope
  Signal Editor : SignalEditorBlockLib/Signal Editor  FileName=A_P_8.mat  ActiveScenario=Scenario  ActiveSignal=A_P_8  IsBus=off  OutputBusObjectStr=Bus: BusObject  SampleTime=0  ZeroCross=off  OutputAfterFinalValue=Setting to zero  Unit=inherit  PreserveSignalName=on  ApplySigPropsToAllScenarios=on
  Signal Editor1 : SignalEditorBlockLib/Signal Editor  FileName=A_T_8.mat  ActiveScenario=Scenario  ActiveSignal=A_T_8  IsBus=off  OutputBusObjectStr=Bus: BusObject  SampleTime=0  ZeroCross=off  OutputAfterFinalValue=Setting to zero  Unit=inherit  PreserveSignalName=on  ApplySigPropsToAllScenarios=on
  Sine Wave : Sin  Amplitude=Vdisp/2  Bias=Vo + (Vdisp/2)  Frequency=omega  Phase=pi/2-(14*pi/9)  SampleTime=0
  T side area : Scope
  Tank Side Flow Rate : MATLAB Function  TreatAsAtomicUnit=on
  Vc : Scope
  Vc_dot : Scope
  P8 Flow Out : Outport
  P8 Flow In : Outport  Port=2
  P8 Eout : Outport  Port=3
  wires:
  Signal Editor/1 -> P side area/1, [A_P]
  [A_P] -> Pressure Side Flow Rate/1(A_P)
  Pressure Side Flow Rate/1(Q_P) -> Q_P/1, [Q_P]
  Tank Side Flow Rate/1(Q_T) -> Q_T/1, [Q_T]
  Constant4/1 -> Tank Side Flow Rate/5(rho), Pressure Side Flow Rate/5(rho)
  Constant2/1 -> Pressure Side Flow Rate/3(P_P)
  [Q_P] -> Compressibility Function/3(Q_P)
  Signal Editor1/1 -> [A_T], T side area/1  "A_T"
  [A_T] -> Tank Side Flow Rate/1(A_T)
  Constant1/1 -> Compressibility Function/4(beta)
  [Pc] -> Pressure Side Flow Rate/2(Pc), Tank Side Flow Rate/2(Pc)
  [Vc_dot] -> Compressibility Function/1(Vc_dot)
  [Q_T] -> Compressibility Function/2(Q_T)
  Compressibility Function/1(Pc_dot) -> Integrator/1  "Pc_dot"
  [Vc] -> Compressibility Function/5(Vc)
  Sine Wave/1 -> [Vc], Vc/1, Derivative/1  "Vc"
  Integrator/1 -> [Pc], Scope/1  "Pc"
  Constant3/1 -> Tank Side Flow Rate/4(Cd), Pressure Side Flow Rate/4(Cd)
  Derivative/1 -> Vc_dot/1, [Vc_dot]  "Vc_dot"
  Constant5/1 -> Tank Side Flow Rate/3(P_T)
  [Q_P] -> P8 Flow Out/1
  [Eout] -> P8 Eout/1
  [Q_T] -> P8 Flow In/1
  [Pc] -> Qleak/1(Pc)
  [Eout] -> Divide/1
  Full Throttling Loss (Pressure Side)/1(" E_ftlps") -> [Eftlps]
  Full Throttling Loss (Tank Side)/1(" E_ftlts") -> [Eftlts]
  [Eftlts] -> Add1/5
  [Ehbl] -> Add1/6
  [Q_T] -> Full Throttling Loss (Tank Side)/3(Q_T)
  [Pc] -> Full Throttling Loss (Pressure Side)/1(Pc)
  [Pc] -> Full Throttling Loss (Tank Side)/1(Pc)
  [Vc] -> Frictional Energy Loss/2(Vc)
  [Vc_dot] -> Frictional Energy Loss/1(Vc_dot)
  [Pc] -> Hydrostatic Bearing Loss/1(Pc)
  Constant/1 -> Full Throttling Loss (Pressure Side)/2(P_P)
  [Q_P] -> Full Throttling Loss (Pressure Side)/3(Q_P)
  [Q_P] -> Product/2
  [Efric] -> Add1/2
  Constant6/1 -> Full Throttling Loss (Tank Side)/2(P_T)
  [Ein] -> Divide/2
  Divide/1 -> Gain/1
  Frictional Energy Loss/1(Efric) -> [Efric]
  Product/1 -> Integrator1/1, Output Power/1  "Pout"
  Constant7/1 -> Product/1
  Hydrostatic Bearing Loss/1(Ehbl) -> [Ehbl]
  Gain/1 -> Display/1
  Qleak/1(Eleak) -> [Eleak]
  Integrator1/1 -> Output Energy/1, Add1/1, [Eout]  "Eout"
  [Eftlps] -> Add1/3
  [Eleak] -> Add1/4
  Add1/1 -> [Ein], Input Energy/1

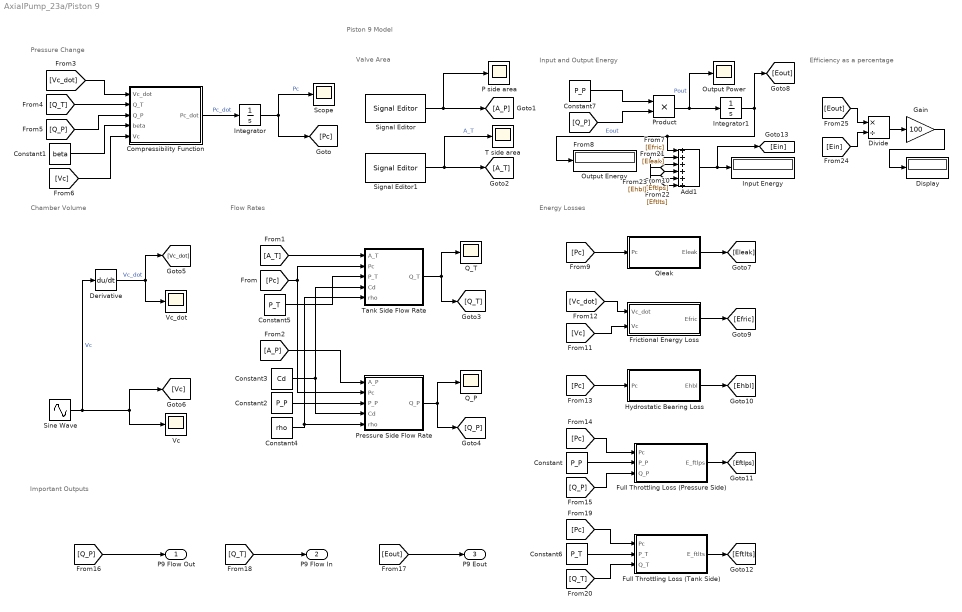
== system AxialPump_23a/Piston 9 ==
  note: Important Outputs
  note: Pressure Change
  note: Chamber Volume
  note: Valve Area
  note: Flow Rates
  note: Piston 9 Model
      | ​
  note: Energy Losses
  note: Efficiency as a percentage
  note: Input and Output Energy
  Add1 : Sum  Inputs=++++++
  Compressibility Function : MATLAB Function  TreatAsAtomicUnit=on
  Constant : Constant  Value=P_P
  Constant1 : Constant  Value=beta
  Constant2 : Constant  Value=P_P
  Constant3 : Constant  Value=Cd
  Constant4 : Constant  Value=rho
  Constant5 : Constant  Value=P_T
  Constant6 : Constant  Value=P_T
  Constant7 : Constant  Value=P_P
  Derivative : Derivative
  Display : Display
  Divide : Product  Inputs=*/
  Frictional Energy Loss : Subsystem
  Full Throttling Loss (Pressure Side) : Subsystem
  Full Throttling Loss (Tank Side) : Subsystem
  Gain : Gain  Gain=100
  Hydrostatic Bearing Loss : Subsystem
  Input Energy : Display
  Integrator : Integrator  InitialCondition=P_T
  Integrator1 : Integrator
  Output Energy : Display
  Output Power : Scope
  P side area : Scope
  Pressure Side Flow Rate : MATLAB Function  TreatAsAtomicUnit=on
  Product : Product
  Q_P : Scope
  Q_T : Scope
  Qleak : Subsystem
  Scope : Scope
  Signal Editor : SignalEditorBlockLib/Signal Editor  FileName=A_P_9.mat  ActiveScenario=Scenario  ActiveSignal=A_P_9  IsBus=off  OutputBusObjectStr=Bus: BusObject  SampleTime=0  ZeroCross=off  OutputAfterFinalValue=Setting to zero  Unit=inherit  PreserveSignalName=on  ApplySigPropsToAllScenarios=on
  Signal Editor1 : SignalEditorBlockLib/Signal Editor  FileName=A_T_9.mat  ActiveScenario=Scenario  ActiveSignal=A_T_9  IsBus=off  OutputBusObjectStr=Bus: BusObject  SampleTime=0  ZeroCross=off  OutputAfterFinalValue=Setting to zero  Unit=inherit  PreserveSignalName=on  ApplySigPropsToAllScenarios=on
  Sine Wave : Sin  Amplitude=Vdisp/2  Bias=Vo + (Vdisp/2)  Frequency=omega  Phase=pi/2-(16*pi/9)  SampleTime=0
  T side area : Scope
  Tank Side Flow Rate : MATLAB Function  TreatAsAtomicUnit=on
  Vc : Scope
  Vc_dot : Scope
  P9 Flow Out : Outport
  P9 Flow In : Outport  Port=2
  P9 Eout : Outport  Port=3
  wires:
  Signal Editor/1 -> P side area/1, [A_P]
  [A_P] -> Pressure Side Flow Rate/1(A_P)
  Pressure Side Flow Rate/1(Q_P) -> Q_P/1, [Q_P]
  Tank Side Flow Rate/1(Q_T) -> Q_T/1, [Q_T]
  Constant4/1 -> Tank Side Flow Rate/5(rho), Pressure Side Flow Rate/5(rho)
  Constant2/1 -> Pressure Side Flow Rate/3(P_P)
  [Q_P] -> Compressibility Function/3(Q_P)
  Signal Editor1/1 -> [A_T], T side area/1  "A_T"
  [A_T] -> Tank Side Flow Rate/1(A_T)
  Constant1/1 -> Compressibility Function/4(beta)
  [Pc] -> Pressure Side Flow Rate/2(Pc), Tank Side Flow Rate/2(Pc)
  [Vc_dot] -> Compressibility Function/1(Vc_dot)
  [Q_T] -> Compressibility Function/2(Q_T)
  Compressibility Function/1(Pc_dot) -> Integrator/1  "Pc_dot"
  [Vc] -> Compressibility Function/5(Vc)
  Sine Wave/1 -> [Vc], Vc/1, Derivative/1  "Vc"
  Integrator/1 -> [Pc], Scope/1  "Pc"
  Constant3/1 -> Tank Side Flow Rate/4(Cd), Pressure Side Flow Rate/4(Cd)
  Derivative/1 -> Vc_dot/1, [Vc_dot]  "Vc_dot"
  Constant5/1 -> Tank Side Flow Rate/3(P_T)
  [Q_P] -> P9 Flow Out/1
  [Eout] -> P9 Eout/1
  [Q_T] -> P9 Flow In/1
  [Pc] -> Qleak/1(Pc)
  [Eout] -> Divide/1
  Full Throttling Loss (Pressure Side)/1(" E_ftlps") -> [Eftlps]
  Full Throttling Loss (Tank Side)/1(" E_ftlts") -> [Eftlts]
  [Eftlts] -> Add1/5
  [Ehbl] -> Add1/6
  [Q_T] -> Full Throttling Loss (Tank Side)/3(Q_T)
  [Pc] -> Full Throttling Loss (Pressure Side)/1(Pc)
  [Pc] -> Full Throttling Loss (Tank Side)/1(Pc)
  [Vc] -> Frictional Energy Loss/2(Vc)
  [Vc_dot] -> Frictional Energy Loss/1(Vc_dot)
  [Pc] -> Hydrostatic Bearing Loss/1(Pc)
  Constant/1 -> Full Throttling Loss (Pressure Side)/2(P_P)
  [Q_P] -> Full Throttling Loss (Pressure Side)/3(Q_P)
  [Q_P] -> Product/2
  [Efric] -> Add1/2
  Constant6/1 -> Full Throttling Loss (Tank Side)/2(P_T)
  [Ein] -> Divide/2
  Divide/1 -> Gain/1
  Frictional Energy Loss/1(Efric) -> [Efric]
  Product/1 -> Integrator1/1, Output Power/1  "Pout"
  Constant7/1 -> Product/1
  Hydrostatic Bearing Loss/1(Ehbl) -> [Ehbl]
  Gain/1 -> Display/1
  Qleak/1(Eleak) -> [Eleak]
  Integrator1/1 -> Output Energy/1, Add1/1, [Eout]  "Eout"
  [Eftlps] -> Add1/3
  [Eleak] -> Add1/4
  Add1/1 -> [Ein], Input Energy/1

== system AxialPump_23a/Piston 1/Eleak ==
  Pc : Inport
  Constant : Constant  Value=P_T
  Constant1 : Constant  Value=d_cyl
  Constant2 : Constant  Value=c
  Constant3 : Constant  Value=meu
  Constant4 : Constant  Value=S
  Display : Display
  Integrator2 : Integrator
  MATLAB Function : MATLAB Function  TreatAsAtomicUnit=on
  Product1 : Product
  Eleak : Outport
  wires:
  Constant/1 -> MATLAB Function/2(P_T)
  Constant1/1 -> MATLAB Function/3(d_cyl)
  Constant2/1 -> MATLAB Function/4(c)
  Constant3/1 -> MATLAB Function/5(meu)
  Constant4/1 -> MATLAB Function/6(S)
  Pc/1 -> MATLAB Function/1(Pc), Product1/2
  MATLAB Function/1(Qleak) -> Product1/1
  Integrator2/1 -> Display/1, Eleak/1
  Product1/1 -> Integrator2/1  "Pleakage"

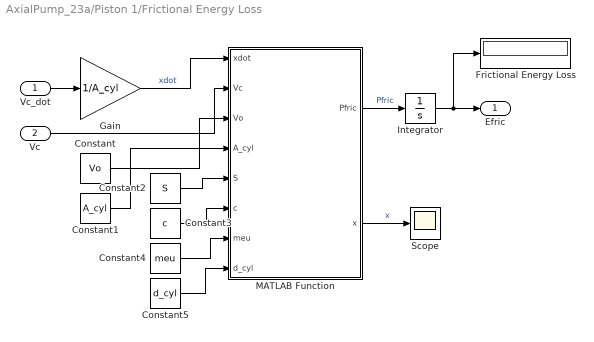
== system AxialPump_23a/Piston 1/Frictional Energy Loss ==
  Vc_dot : Inport
  Vc : Inport  Port=2
  Constant : Constant  Value=Vo
  Constant1 : Constant  Value=A_cyl
  Constant2 : Constant  Value=S
  Constant3 : Constant  Value=c
  Constant4 : Constant  Value=meu
  Constant5 : Constant  Value=d_cyl
  Frictional Energy Loss : Display
  Gain : Gain  Gain=1/A_cyl
  Integrator : Integrator
  MATLAB Function : MATLAB Function  TreatAsAtomicUnit=on
  Scope : Scope
  Efric : Outport
  wires:
  Integrator/1 -> Frictional Energy Loss/1, Efric/1
  Vc_dot/1 -> Gain/1
  Gain/1 -> MATLAB Function/1(xdot)  "xdot"
  MATLAB Function/1(Pfric) -> Integrator/1  "Pfric"
  MATLAB Function/2(x) -> Scope/1  "x"
  Vc/1 -> MATLAB Function/2(Vc)
  Constant/1 -> MATLAB Function/3(Vo)
  Constant1/1 -> MATLAB Function/4(A_cyl)
  Constant2/1 -> MATLAB Function/5(S)
  Constant3/1 -> MATLAB Function/6(c)
  Constant4/1 -> MATLAB Function/7(meu)
  Constant5/1 -> MATLAB Function/8(d_cyl)

== system AxialPump_23a/Piston 1/Full Throttling Loss (Pressure Side) ==
  Pc : Inport
  P_P : Inport  Port=2
  Q_P : Inport  Port=3
  Display : Display
  Integrator : Integrator
  MATLAB Function : MATLAB Function  TreatAsAtomicUnit=on
  Scope : Scope
  " E_ftlps" : Outport
  wires:
  MATLAB Function/1(P_ftlps) -> Scope/1, Integrator/1
  Integrator/1 -> Display/1, " E_ftlps"/1  "E_ftlps"
  Pc/1 -> MATLAB Function/1(Pc)
  P_P/1 -> MATLAB Function/2(P_P)
  Q_P/1 -> MATLAB Function/3(Q_P)

== system AxialPump_23a/Piston 1/Full Throttling Loss (Tank Side) ==
  Pc : Inport
  P_T : Inport  Port=2
  Q_T : Inport  Port=3
  Display : Display
  Integrator : Integrator
  MATLAB Function : MATLAB Function  TreatAsAtomicUnit=on
  Scope : Scope
  " E_ftlts" : Outport
  wires:
  MATLAB Function/1(P_ftlts) -> Scope/1, Integrator/1
  Integrator/1 -> Display/1, " E_ftlts"/1  "E_ftlts"
  Pc/1 -> MATLAB Function/2(Pc)
  P_T/1 -> MATLAB Function/1(P_T)
  Q_T/1 -> MATLAB Function/3(Q_T)

== system AxialPump_23a/Piston 1/Hydrostatic Bearing Loss ==
  Pc : Inport
  Constant : Constant  Value=Cd
  Constant1 : Constant  Value=r2_r1
  Constant2 : Constant  Value=r1
  Constant3 : Constant  Value=do
  Constant4 : Constant  Value=d_cyl
  Constant5 : Constant  Value=rho
  Display : Display
  Integrator : Integrator
  MATLAB Function : MATLAB Function  TreatAsAtomicUnit=on
  Product : Product
  Ehbl : Outport
  wires:
  Constant1/1 -> MATLAB Function/2(r2_r1)
  Constant/1 -> MATLAB Function/6(Cd)
  Constant4/1 -> MATLAB Function/5(d_cyl)
  Constant3/1 -> MATLAB Function/4(do)
  Constant2/1 -> MATLAB Function/3(r1)
  Pc/1 -> Product/2, MATLAB Function/7(Pc)
  MATLAB Function/1(Qhbl) -> Product/1
  Product/1 -> Integrator/1  "Phbl"
  Integrator/1 -> Display/1, Ehbl/1
  Constant5/1 -> MATLAB Function/1(rho)

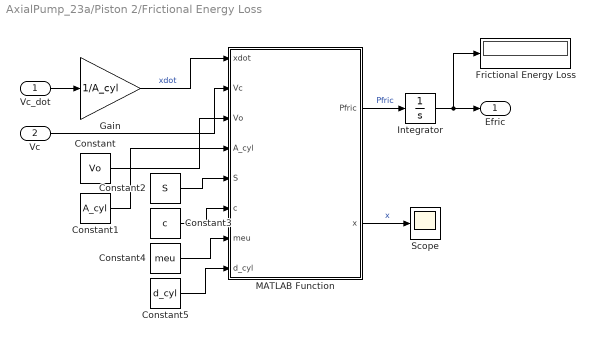
== system AxialPump_23a/Piston 2/Frictional Energy Loss ==
  Vc_dot : Inport
  Vc : Inport  Port=2
  Constant : Constant  Value=Vo
  Constant1 : Constant  Value=A_cyl
  Constant2 : Constant  Value=S
  Constant3 : Constant  Value=c
  Constant4 : Constant  Value=meu
  Constant5 : Constant  Value=d_cyl
  Frictional Energy Loss : Display
  Gain : Gain  Gain=1/A_cyl
  Integrator : Integrator
  MATLAB Function : MATLAB Function  TreatAsAtomicUnit=on
  Scope : Scope
  Efric : Outport
  wires:
  Integrator/1 -> Frictional Energy Loss/1, Efric/1
  Vc_dot/1 -> Gain/1
  Gain/1 -> MATLAB Function/1(xdot)  "xdot"
  MATLAB Function/1(Pfric) -> Integrator/1  "Pfric"
  MATLAB Function/2(x) -> Scope/1  "x"
  Vc/1 -> MATLAB Function/2(Vc)
  Constant/1 -> MATLAB Function/3(Vo)
  Constant1/1 -> MATLAB Function/4(A_cyl)
  Constant2/1 -> MATLAB Function/5(S)
  Constant3/1 -> MATLAB Function/6(c)
  Constant4/1 -> MATLAB Function/7(meu)
  Constant5/1 -> MATLAB Function/8(d_cyl)

== system AxialPump_23a/Piston 2/Full Throttling Loss (Pressure Side) ==
  Pc : Inport
  P_P : Inport  Port=2
  Q_P : Inport  Port=3
  Display : Display
  Integrator : Integrator
  MATLAB Function : MATLAB Function  TreatAsAtomicUnit=on
  Scope : Scope
  " E_ftlps" : Outport
  wires:
  MATLAB Function/1(P_ftlps) -> Scope/1, Integrator/1
  Integrator/1 -> Display/1, " E_ftlps"/1  "E_ftlps"
  Pc/1 -> MATLAB Function/1(Pc)
  P_P/1 -> MATLAB Function/2(P_P)
  Q_P/1 -> MATLAB Function/3(Q_P)
